simulink model "MicroMouseTemplate_2025"  (R2024b)
settings: Solver=FixedStepAuto  StartTime=0.0  StopTime=inf  FixedStep=0.01  RelTol=1e-3  EnableMultiTasking=on
PreLoadFcn:
  | runMeFirst
settings Model: STM32="{\"DigitalPortWrite\":[{\"ID\":\"MicroMouseTemplate_2025:4:4\"},{\"ID\":\"MicroMouseTemplate_2025:4:6\"},{\"ID\":\"MicroMouseTemplate_2025:4:7\"},{\"ID\":\"MicroMouseTemplate_2025:4:8\"},{\"ID\":\"MicroMouseTemplate_2025:4:2501\"},{\"ID\":\"MicroMouseTemplate_2025:4:2502\"}],\"DigitalPortRead\":[{\"ID\":\"MicroMouseTemplate_2025:9:3\"},{\"ID\":\"MicroMouseTemplate_2025:9:4\"},{\"ID\":\"MicroMouseTemplate_2025:9:2497\"},{\"ID\":\"MicroMouseTemplate_2025:9:2498\"}],\"I2CControllerRead\":[{\"ID\":\"MicroMouseTemplate_2025:10:2496\"},{\"ID\":\"MicroMouseTemplate_2025:10:2519\"},{\"ID\":\"MicroMouseTemplate_2025:10:2520\"},{\"ID\":\"MicroMouseTemplate_2025:10:2523\"},{\"ID\":\"MicroMouseTemplate_2025:10:2524\"},{\"ID\":\"MicroMouseTemplate_2025:10:2525\"},{\"ID\":\"MicroMouseTemplate_2025:10:2531\"}],\"I2CControllerWrite\":[{\"ID\":\"MicroMouseTemplate_2025:10:2509\"},{\"ID\":\"MicroMouseTemplate_2025:10:2510\"},{\"ID\":\"MicroMouseTemplate_2025:10:2511\"},{\"ID\":\"MicroMouseTemplate_2025:10:2512\"}]}"  SimulationMode=external  Creator=JesseJabezArendse  LastModifiedBy=JesseJabezArendse
settings SolverCC: AutoInsertRateTranBlk=on
settings OptimizationCC: OptimizeBlockIOStorage=off  BufferReuse=off  ReuseModelBlockBuffer=off  GlobalBufferReuse=off  ExpressionFolding=off  EnableMemcpy=off  PassReuseOutputArgsAs=Individual arguments  LocalBlockOutputs=off  ZeroExternalMemoryAtStartup=off  ZeroInternalMemoryAtStartup=off  MaxStackSize=512  OptimizeDataStoreBuffers=off  BusAssignmentInplaceUpdate=off  OptimizationLevel=level0  OptimizationCustomize=off  EfficientTunableParamExpr=on
settings DebuggingCC: ParameterTunabilityLossMsg=error
settings HardwareCC: ProdBitPerPointer=32  ProdBitPerSizeT=32  ProdBitPerPtrDiffT=32  ProdLargestAtomicInteger=Long  ProdLargestAtomicFloat=Double  ProdWordSize=32  ProdLongLongMode=on  ProdHWDeviceType=ARM Compatible->ARM Cortex-M
settings ModelReferenceCC: UpdateModelReferenceTargets=IfOutOfDate  EnableParallelModelReferenceBuilds=on
settings SFSimCC: MATLABDynamicMemAlloc=off  SimHardwareAcceleration=native
settings RTWCC: Description=Embedded Coder  SystemTargetFile=ert.tlc  HardwareBoard=STM32L4xx Based  TemplateMakefile=ert_default_tmf  CustomHeaderCode="#include \"MicroMouseProgramming\\Core\\Inc\\main.h\""  CustomSource=MicroMouseProgramming\Core\Src\main.c  Toolchain=GNU Tools for ARM Embedded Processors  BuildConfiguration=Debug
settings RTWCC: CustomInclude=|
  | MicroMouseProgramming\Core\Src
  | MicroMouseProgramming\Core\Inc
settings CodeAppCC: ForceParamTrailComments=on  IgnoreCustomStorageClasses=off  OperatorAnnotations=on  SimulinkDataObjDesc=on  SFDataObjDesc=on  InsertBlockDesc=on
settings ERTTargetCC: TargetLangStandard=C99 (ISO)  CodeReplacementLibrary=ARM Cortex-M,GNU C99 extensions  ExtModeTransport=3  ExtModeStaticAlloc=on  ExtModeStaticAllocSize=2048  ExtModeMexFile=ext_xcp  ExtModeIntrfLevel=Level2 - Open  InlinedParameterPlacement=Hierarchical

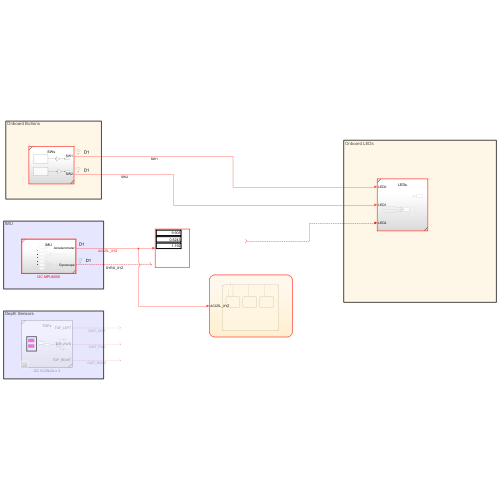
[thumbnail: Simulink's stored preview of the top-level diagram]
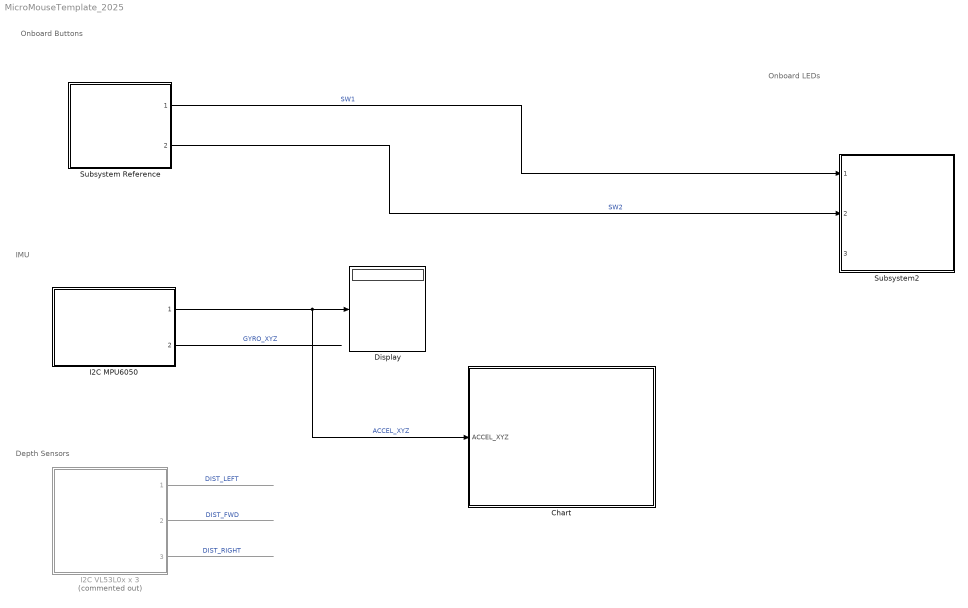
== system MicroMouseTemplate_2025 ==
  note: Onboard Buttons
  note: Onboard LEDs
  note: IMU
  note: Depth Sensors
  Chart : Stateflow chart  TreatAsAtomicUnit=on
  Display : Display
  I2C MPU6050 : Subsystem  TreatAsAtomicUnit=on  ReferencedSubsystem=IMU
  I2C VL53L0x x 3 : Subsystem  Commented=on  ReferencedSubsystem=TOFs
  Subsystem Reference : Subsystem  ReferencedSubsystem=SWs
  Subsystem2 : Subsystem  ReferencedSubsystem=LEDs
  wires:
  Subsystem Reference/2 -> Subsystem2/2  "SW2"
  ? -> Subsystem2/3
  Subsystem Reference/1 -> Subsystem2/1  "SW1"
  I2C MPU6050/1 -> Chart/1(ACCEL_XYZ), Display/1  "ACCEL_XYZ"
  I2C MPU6050/2 -> ?  "GYRO_XYZ"
  I2C VL53L0x x 3/1 -> ?  "DIST_LEFT"
  I2C VL53L0x x 3/2 -> ?  "DIST_FWD"
  I2C VL53L0x x 3/3 -> ?  "DIST_RIGHT"

== stateflow chart MicroMouseTemplate_2025/Chart ==
  state LED_IND
    note: [ACCEL_XYZ(2) >= 9]
    state X
    state Y
    state Z
    LED_IND -> X [order 1] : [ACCEL_XYZ(1) >= 9]
    LED_IND -> Y [order 2]
    LED_IND -> Z [order 3] : [ACCEL_XYZ(3) >= 9]
    (default) -> X
  (default) -> LED_IND
  data: ACCEL_XYZ input
